simulink model "Week3_Problem2"  (R2020b)
settings: Solver=FixedStepAuto  StartTime=0.0  StopTime=10.0  FixedStep=.1  RelTol=1e-3  EnableMultiTasking=on
undefined symbols (not defined in the file): DiscIntNeverNeededParam
libraries: simulink x1
settings Model: Creator=Akshay A H  LastModifiedBy=Akshay A H

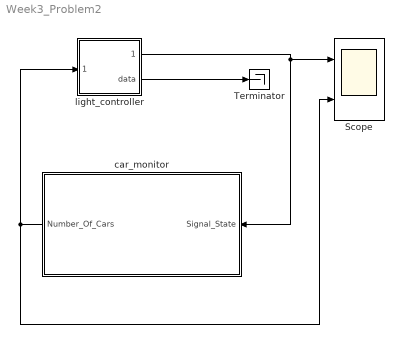
== system Week3_Problem2 ==
  Scope : Scope  NumInputPorts=2
  Terminator : Terminator
  car_monitor : Subsystem
  light_controller : Stateflow chart  TreatAsAtomicUnit=on
  wires:
  light_controller/2(data) -> Terminator/1
  light_controller/1(data1) -> car_monitor/1(Signal_State), Scope/1
  car_monitor/1(Number_Of_Cars) -> light_controller/1(Number_Of_Cars), Scope/2

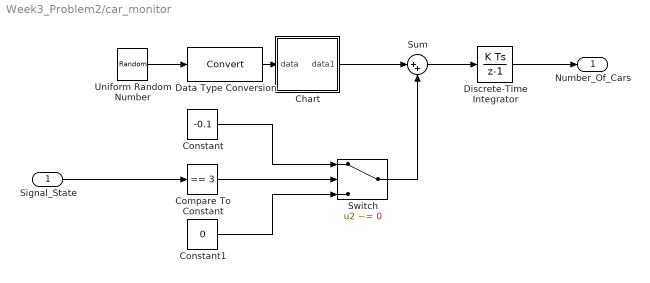
== system Week3_Problem2/car_monitor ==
  Signal_State : Inport
  Chart : Stateflow chart  TreatAsAtomicUnit=on
  Compare To Constant : simulink/Logic and Bit Operations/Compare To Constant  relop===  const=3  OutDataTypeStr=boolean  ZeroCross=off
  Constant : Constant  Value=-0.1
  Constant1 : Constant  Value=0
  Data Type Conversion : DataTypeConversion
  Discrete-Time Integrator : DiscreteIntegrator  SampleTime=-1  LimitOutput=on  ICPrevOutput=DiscIntNeverNeededParam  ICPrevScaledInput=DiscIntNeverNeededParam
  Sum : Sum  Inputs=|++
  Switch : Switch  Criteria=u2 ~= 0  ZeroCross=off
  Uniform Random Number : UniformRandomNumber  Minimum=0  Maximum=100  Seed=177836  SampleTime=0
  Number_Of_Cars : Outport
  wires:
  Compare To Constant/1 -> Switch/2
  Switch/1 -> Sum/2
  Data Type Conversion/1 -> Chart/1(data)
  Uniform Random Number/1 -> Data Type Conversion/1
  Chart/1(data1) -> Sum/1
  Constant/1 -> Switch/1
  Constant1/1 -> Switch/3
  Signal_State/1 -> Compare To Constant/1
  Sum/1 -> Discrete-Time Integrator/1
  Discrete-Time Integrator/1 -> Number_Of_Cars/1

== stateflow chart Week3_Problem2/car_monitor/Chart ==
  (default) -> (junction 1) : {data1 = data>98;}
  data: data input; data1 output

== stateflow chart Week3_Problem2/light_controller ==
  state stop
    data1 = red;
    data=green;
  state stopForTraffic
    data1=red;
    data=green;
  state stopToGo
    data1=red;
    data=yellow;
  state goToStop
    data1=yellow;
    data=red;
  state go
    data1 = green;
    data=red;
  (default) -> stop
  stop -> stopForTraffic : after(20,tick)
  stopForTraffic -> stopToGo : [Number_Of_Cars]
  goToStop -> stop : after(3,tick)
  stopToGo -> go : after(3,tick)
  go -> goToStop : after(10,tick)
  data: data1 output; data output; Number_Of_Cars input
